simulink model "STFTDiffWindowSizes"  (R2021b)
settings: Solver=VariableStepAuto  StartTime=0.0  StopTime=2048*15/fs  RelTol=1e-3
InitFcn:
  | f = 12.288e6;
  | fs = 153.6e6;
  | N1 = 256;
  | N2 = 512;
  | N3 = 1024;
  | N4 = 2048;
  | N5 = 4096;
  | n1 = 0:N1-1;
  | n2 = 0:N2-1;
  | n3 = 0:N3-1;
  | n4 = 0:N4-1;
  | n5 = 0:N5-1;
  | Hamming1 = 0.54 - 0.46 * cos(2*pi*n1/N1);
  | Hamming2 = 0.54 - 0.46 * cos(2*pi*n2/N2);
  | Hamming3 = 0.54 - 0.46 * cos(2*pi*n3/N3);
  | Hamming4 = 0.54 - 0.46 * cos(2*pi*n4/N4);
  | Hamming5 = 0.54 - 0.46 * cos(2*pi*n5/N5);
  | Hanning1 = 0.5 * (1 + cos(2*pi*n1/N1));
  | Hanning2 = 0.5 * (1 + cos(2*pi*n2/N2));
  | Hanning3 = 0.5 * (1 + cos(2*pi*n3/N3));
  | Hanning4 = 0.5 * (1 + cos(2*pi*n4/N4));
  | Hanning5 = 0.5 * (1 + cos(2*pi*n5/N5));
  | Norm_Ham1 = sum(Hamming1);
  | Norm_Ham2 = sum(Hamming2);
  | Norm_Ham3 = sum(Hamming3);
  | Norm_Ham4 = sum(Hamming4);
  | Norm_Ham5 = sum(Hamming5);
  | Norm_Han1 = sum(Hanning1);
  | Norm_Han2 = sum(Hanning2);
  | Norm_Han3 = sum(Hanning3);
  | Norm_Han4 = sum(Hanning4);
  | Norm_Han5 = sum(Hanning5);
undefined symbols (not defined in the file): AXI4, Lite, Norm_Ham, Norm_Han
libraries: hdlBasic x321, hdlDSPIP x10, hdlsllib x1, vmcUtilities x1
(part 3 of 3)

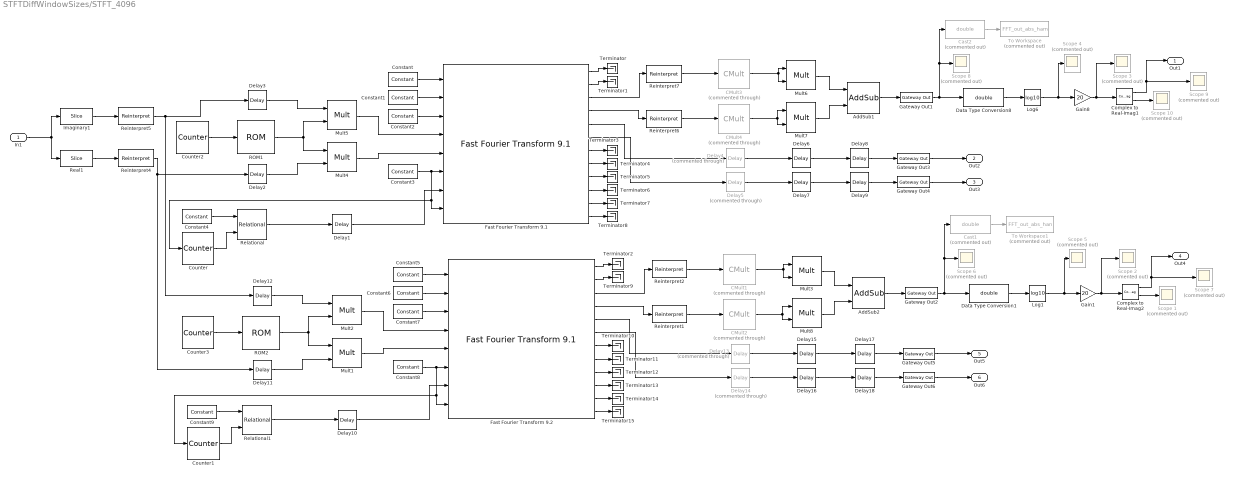
== system STFTDiffWindowSizes/STFT_4096 ==
  In1 : Inport
  AddSub1 : hdlBasic/AddSub  mode=Addition  use_carryin=off  use_carryout=off  en=off  latency=1  precision=User Defined  arith_type=Unsigned  n_bits=32  bin_pt=30  quantization=Truncate  overflow=Saturate  use_behavioral_HDL=off  hw_selection=Fabric  pipelined=off  XmcBlockStatus=1  maskContainerNames=tabcontainer1  block_type=addsub  block_config=sysgen:Addsub_config
  AddSub2 : hdlBasic/AddSub  mode=Addition  use_carryin=off  use_carryout=off  en=off  latency=1  precision=User Defined  arith_type=Unsigned  n_bits=32  bin_pt=30  quantization=Truncate  overflow=Saturate  use_behavioral_HDL=off  hw_selection=Fabric  pipelined=off  XmcBlockStatus=1  maskContainerNames=tabcontainer1  block_type=addsub  block_config=sysgen:Addsub_config
  CMult1 : hdlBasic/CMult  Commented=through  const=1/Norm_Han  gui_display_data_type=Fixed-point  const_n_bits=32  const_bin_pt=31  float_type=Single  exp_bits=8  fraction_bits=24  en=off  latency=3  precision=User Defined  arith_type=Unsigned  n_bits=32  bin_pt=31  quantization=Truncate  overflow=Saturate  use_behavioral_HDL=off  mem_type=Distributed RAM  pipeline=off  XmcBlockStatus=1  maskContainerNames=tabcontainer1  block_type=cmult  block_config=sysgen:CMult_config
      settings: infoedit=[]
  CMult2 : hdlBasic/CMult  Commented=through  const=1/Norm_Han  gui_display_data_type=Fixed-point  const_n_bits=32  const_bin_pt=31  float_type=Single  exp_bits=8  fraction_bits=24  en=off  latency=3  precision=User Defined  arith_type=Unsigned  n_bits=32  bin_pt=31  quantization=Truncate  overflow=Saturate  use_behavioral_HDL=off  mem_type=Distributed RAM  pipeline=off  XmcBlockStatus=1  maskContainerNames=tabcontainer1  block_type=cmult  block_config=sysgen:CMult_config
      settings: infoedit=[]
  CMult3 : hdlBasic/CMult  Commented=through  const=1/Norm_Ham  gui_display_data_type=Fixed-point  const_n_bits=32  const_bin_pt=31  float_type=Single  exp_bits=8  fraction_bits=24  en=off  latency=3  precision=User Defined  arith_type=Unsigned  n_bits=32  bin_pt=31  quantization=Truncate  overflow=Saturate  use_behavioral_HDL=off  mem_type=Distributed RAM  pipeline=off  XmcBlockStatus=1  maskContainerNames=tabcontainer1  block_type=cmult  block_config=sysgen:CMult_config
      settings: infoedit=[]
  CMult4 : hdlBasic/CMult  Commented=through  const=1/Norm_Ham  gui_display_data_type=Fixed-point  const_n_bits=32  const_bin_pt=31  float_type=Single  exp_bits=8  fraction_bits=24  en=off  latency=3  precision=User Defined  arith_type=Unsigned  n_bits=32  bin_pt=31  quantization=Truncate  overflow=Saturate  use_behavioral_HDL=off  mem_type=Distributed RAM  pipeline=off  XmcBlockStatus=1  maskContainerNames=tabcontainer1  block_type=cmult  block_config=sysgen:CMult_config
      settings: infoedit=[]
  Cast1 : DataTypeConversion  Commented=on  OutDataTypeStr=double
  Cast2 : DataTypeConversion  Commented=on  OutDataTypeStr=double
  Complex to Real-Imag1 : ComplexToRealImag
  Complex to Real-Imag2 : ComplexToRealImag
  Constant : hdlBasic/Constant  const=0  gui_display_data_type=Fixed-point  arith_type=Unsigned  n_bits=12  bin_pt=0  preci_type=Single  exp_width=8  frac_width=24  explicit_period=on  period=1/fs  XmcBlockStatus=1  maskContainerNames=tabcontainer1  block_type=constant  block_config=sysgen:Constant_config
  Constant1 : hdlBasic/Constant  const=0  gui_display_data_type=Fixed-point  arith_type=Unsigned  n_bits=1  bin_pt=0  preci_type=Single  exp_width=8  frac_width=24  explicit_period=on  period=1/fs  XmcBlockStatus=1  maskContainerNames=tabcontainer1  block_type=constant  block_config=sysgen:Constant_config
  Constant2 : hdlBasic/Constant  const=0  gui_display_data_type=Boolean  arith_type=Boolean  n_bits=1  bin_pt=0  preci_type=Single  exp_width=8  frac_width=24  explicit_period=on  period=1/fs  XmcBlockStatus=1  maskContainerNames=tabcontainer1  block_type=constant  block_config=sysgen:Constant_config
  Constant3 : hdlBasic/Constant  const=1  gui_display_data_type=Boolean  arith_type=Boolean  n_bits=1  bin_pt=0  preci_type=Single  exp_width=8  frac_width=24  explicit_period=on  period=1/fs  XmcBlockStatus=1  maskContainerNames=tabcontainer1  block_type=constant  block_config=sysgen:Constant_config
  Constant4 : hdlBasic/Constant  const=N5-1  gui_display_data_type=Fixed-point  arith_type=Unsigned  n_bits=12  bin_pt=0  preci_type=Single  exp_width=8  frac_width=24  explicit_period=on  period=1/fs  XmcBlockStatus=1  maskContainerNames=tabcontainer1  block_type=constant  block_config=sysgen:Constant_config
  Constant5 : hdlBasic/Constant  const=0  gui_display_data_type=Fixed-point  arith_type=Unsigned  n_bits=12  bin_pt=0  preci_type=Single  exp_width=8  frac_width=24  explicit_period=on  period=1/fs  XmcBlockStatus=1  maskContainerNames=tabcontainer1  block_type=constant  block_config=sysgen:Constant_config
  Constant6 : hdlBasic/Constant  const=0  gui_display_data_type=Fixed-point  arith_type=Unsigned  n_bits=1  bin_pt=0  preci_type=Single  exp_width=8  frac_width=24  explicit_period=on  period=1/fs  XmcBlockStatus=1  maskContainerNames=tabcontainer1  block_type=constant  block_config=sysgen:Constant_config
  Constant7 : hdlBasic/Constant  const=0  gui_display_data_type=Boolean  arith_type=Boolean  n_bits=1  bin_pt=0  preci_type=Single  exp_width=8  frac_width=24  explicit_period=on  period=1/fs  XmcBlockStatus=1  maskContainerNames=tabcontainer1  block_type=constant  block_config=sysgen:Constant_config
  Constant8 : hdlBasic/Constant  const=1  gui_display_data_type=Boolean  arith_type=Boolean  n_bits=1  bin_pt=0  preci_type=Single  exp_width=8  frac_width=24  explicit_period=on  period=1/fs  XmcBlockStatus=1  maskContainerNames=tabcontainer1  block_type=constant  block_config=sysgen:Constant_config
  Constant9 : hdlBasic/Constant  const=N5-1  gui_display_data_type=Fixed-point  arith_type=Unsigned  n_bits=12  bin_pt=0  preci_type=Single  exp_width=8  frac_width=24  explicit_period=on  period=1/fs  XmcBlockStatus=1  maskContainerNames=tabcontainer1  block_type=constant  block_config=sysgen:Constant_config
  Counter : hdlBasic/Counter  cnt_type=Count limited  cnt_to=N5-1  operation=Up  start_count=0  cnt_by_val=1  arith_type=Unsigned  n_bits=12  bin_pt=0  load_pin=off  rst=off  en=on  explicit_period=Explicit  period=1/fs  use_behavioral_HDL=off  implementation=Fabric  XmcBlockStatus=1  maskContainerNames=group1  block_type=counter  block_config=sysgen:Counter_config
  Counter1 : hdlBasic/Counter  cnt_type=Count limited  cnt_to=N5-1  operation=Up  start_count=0  cnt_by_val=1  arith_type=Unsigned  n_bits=12  bin_pt=0  load_pin=off  rst=off  en=on  explicit_period=Explicit  period=1/fs  use_behavioral_HDL=off  implementation=Fabric  XmcBlockStatus=1  maskContainerNames=group1  block_type=counter  block_config=sysgen:Counter_config
  Counter2 : hdlBasic/Counter  cnt_type=Count limited  cnt_to=N5-1  operation=Up  start_count=0  cnt_by_val=1  arith_type=Unsigned  n_bits=12  bin_pt=0  load_pin=off  rst=off  en=off  explicit_period=Explicit  period=1/fs  use_behavioral_HDL=off  implementation=Fabric  XmcBlockStatus=1  maskContainerNames=group1  block_type=counter  block_config=sysgen:Counter_config
  Counter3 : hdlBasic/Counter  cnt_type=Count limited  cnt_to=N5-1  operation=Up  start_count=0  cnt_by_val=1  arith_type=Unsigned  n_bits=12  bin_pt=0  load_pin=off  rst=off  en=off  explicit_period=Explicit  period=1/fs  use_behavioral_HDL=off  implementation=Fabric  XmcBlockStatus=1  maskContainerNames=group1  block_type=counter  block_config=sysgen:Counter_config
  Data Type Conversion1 : DataTypeConversion  OutDataTypeStr=double  SaturateOnIntegerOverflow=on
  Data Type Conversion8 : DataTypeConversion  OutDataTypeStr=double  SaturateOnIntegerOverflow=on
  Delay{1,6..7,10,15..16} (6 alike) : hdlBasic/Delay  rst=off  en=off  latency=3  reg_retiming=off  XmcBlockStatus=1  maskContainerNames=group1  block_type=delay  block_config=sysgen:Delay_config
  Delay{2..3,8..9,11..12,17..18} (8 alike) : hdlBasic/Delay  rst=off  en=off  latency=1  reg_retiming=off  XmcBlockStatus=1  maskContainerNames=group1  block_type=delay  block_config=sysgen:Delay_config
  Delay{4..5,13..14} (4 alike) : hdlBasic/Delay  Commented=through  rst=off  en=off  latency=3  reg_retiming=off  XmcBlockStatus=1  maskContainerNames=group1  block_type=delay  block_config=sysgen:Delay_config
  Fast Fourier Transform 9.1 : hdlDSPIP/Fast Fourier Transform 9.1   transform_length=4096  target_clock_frequency=200  target_data_throughput=50  implementation_options=pipelined_streaming_io  run_time_configurable_transform_length=off  phase_factor_width=16  scaling_options=scaled  rounding_modes=truncation  aclken=off  aresetn=off  output_ordering=natural_order  cyclic_prefix_insertion=off  throttle_scheme=nonrealtime  xk_index=off  ovflo=off  trim_axipin_name=on  memory_options_data=block_ram  memory_options_phase_factors=block_ram  number_of_stages_using_block_ram_for_data_and_phase_factors=6  memory_options_reorder=block_ram  memory_options_hybrid=off  complex_mult_type=use_mults_resources  butterfly_type=use_luts  simulation_type=hybrid_sim  simulation_model=sysgen:xfftv9_cmodel  data_path_portlist={ 's_axis_data_tdata', 'm_axis_data_tdata', 'm_axis_status_tdata', 'event_fft_overflow' }  channels=1  input_ordering=natural_order  input_width=16  ip_name=Fast Fourier Transform  ip_version=9.1  dsptool_ready=true  ipcore_usecache=true  ipcore_useipmodelcache=true  wrapper_available=true  port_translation_map={ 'aclken' => 'en', 'aresetn' => 'rst'}  data_format=fixed_point  XmcBlockStatus=1  maskContainerNames=tabcontainer1  block_type=xfft_v9_1  block_config=sysgen:rodinimport_config
  Fast Fourier Transform 9.2 : hdlDSPIP/Fast Fourier Transform 9.1   transform_length=4096  target_clock_frequency=200  target_data_throughput=50  implementation_options=pipelined_streaming_io  run_time_configurable_transform_length=off  phase_factor_width=16  scaling_options=scaled  rounding_modes=truncation  aclken=off  aresetn=off  output_ordering=natural_order  cyclic_prefix_insertion=off  throttle_scheme=nonrealtime  xk_index=off  ovflo=off  trim_axipin_name=on  memory_options_data=block_ram  memory_options_phase_factors=block_ram  number_of_stages_using_block_ram_for_data_and_phase_factors=6  memory_options_reorder=block_ram  memory_options_hybrid=off  complex_mult_type=use_mults_resources  butterfly_type=use_luts  simulation_type=hybrid_sim  simulation_model=sysgen:xfftv9_cmodel  data_path_portlist={ 's_axis_data_tdata', 'm_axis_data_tdata', 'm_axis_status_tdata', 'event_fft_overflow' }  channels=1  input_ordering=natural_order  input_width=16  ip_name=Fast Fourier Transform  ip_version=9.1  dsptool_ready=true  ipcore_usecache=true  ipcore_useipmodelcache=true  wrapper_available=true  port_translation_map={ 'aclken' => 'en', 'aresetn' => 'rst'}  data_format=fixed_point  XmcBlockStatus=1  maskContainerNames=tabcontainer1  block_type=xfft_v9_1  block_config=sysgen:rodinimport_config
  Gain1 : Gain  Gain=20
  Gain8 : Gain  Gain=20
  Gateway Out1 : hdlBasic/Gateway Out  inherit_from_input=on  hdl_port=on  rows=1  columns=1  UseAsDAC=off  DACChannel='1'  interface=AXI4-Lite  automatic_assignment=on  address_offset=hex2dec('00')  intf_name=''  intf_description=''  timing_constraint=None  locs_specified=off  LOCs={}  io_standard={}  XmcBlockStatus=1  maskContainerNames=group4  block_type=gatewayout  block_config=sysgen:gateway_out_config  block_width_w=590  block_height_w=620  block_width=620  block_height=750
  Gateway Out2 : hdlBasic/Gateway Out  inherit_from_input=on  hdl_port=on  rows=1  columns=1  UseAsDAC=off  DACChannel='1'  interface=AXI4-Lite  automatic_assignment=on  address_offset=hex2dec('00')  intf_name=''  intf_description=''  timing_constraint=None  locs_specified=off  LOCs={}  io_standard={}  XmcBlockStatus=1  maskContainerNames=group4  block_type=gatewayout  block_config=sysgen:gateway_out_config  block_width_w=590  block_height_w=620  block_width=620  block_height=750
  Gateway Out{3..6} (4 alike) : hdlBasic/Gateway Out  inherit_from_input=off  hdl_port=on  rows=1  columns=1  UseAsDAC=off  DACChannel='1'  interface=AXI4-Lite  automatic_assignment=on  address_offset=hex2dec('00')  intf_name=''  intf_description=''  timing_constraint=None  locs_specified=off  LOCs={}  io_standard={}  XmcBlockStatus=1  maskContainerNames=group4  block_type=gatewayout  block_config=sysgen:gateway_out_config  block_width_w=590  block_height_w=620  block_width=620  block_height=750
  Imaginary1 : hdlBasic/Slice  nbits=16  boolean_output=off  mode=Two Bit Locations  bit1=31  base1=LSB of Input  bit0=16  base0=LSB of Input  XmcBlockStatus=1  maskContainerNames=group1  block_type=slice  block_config=sysgen:Slice_config
  Log1 : Math  Operator=log10  OutputSignalType=complex  SaturateOnIntegerOverflow=on
  Log6 : Math  Operator=log10  OutputSignalType=complex  SaturateOnIntegerOverflow=on
  Mult{1..2,4..5} (4 alike) : hdlBasic/Mult  precision=User Defined  arith_type="Signed  (2's comp)"  n_bits=16  bin_pt=15  quantization=Truncate  overflow=Saturate  en=off  latency=3  use_behavioral_HDL=off  opt=Speed  use_embedded=on  optimum_pipeline=off  pipeline=on  use_rpm=on  placement_style=Triangular  XmcBlockStatus=1  maskContainerNames=group1  block_type=mult  block_config=sysgen:Mult_config
  Mult{3,6..8} (4 alike) : hdlBasic/Mult  precision=User Defined  arith_type=Unsigned  n_bits=32  bin_pt=31  quantization=Truncate  overflow=Saturate  en=off  latency=3  use_behavioral_HDL=off  opt=Speed  use_embedded=on  optimum_pipeline=off  pipeline=on  use_rpm=on  placement_style=Triangular  XmcBlockStatus=1  maskContainerNames=group1  block_type=mult  block_config=sysgen:Mult_config
  ROM1 : hdlBasic/ROM  depth=N5  initVector=Hamming5  distributed_mem=Block RAM  rst=off  init_reg=0  en=off  latency=1  gui_display_data_type=Fixed-point  arith_type=Unsigned  n_bits=16  bin_pt=15  preci_type=Single  exp_width=8  frac_width=24  optimize=Area  use_rpm=on  simulation_type=fast_sim  XmcBlockStatus=1  maskContainerNames=tabcontainer1  block_type=sprom  block_config=sysgen:SPROM_config
  ROM2 : hdlBasic/ROM  depth=N5  initVector=Hanning5  distributed_mem=Block RAM  rst=off  init_reg=0  en=off  latency=1  gui_display_data_type=Fixed-point  arith_type=Unsigned  n_bits=16  bin_pt=15  preci_type=Single  exp_width=8  frac_width=24  optimize=Area  use_rpm=on  simulation_type=fast_sim  XmcBlockStatus=1  maskContainerNames=tabcontainer1  block_type=sprom  block_config=sysgen:SPROM_config
  Real1 : hdlBasic/Slice  nbits=16  boolean_output=off  mode=Two Bit Locations  bit1=15  base1=LSB of Input  bit0=0  base0=LSB of Input  XmcBlockStatus=1  maskContainerNames=group1  block_type=slice  block_config=sysgen:Slice_config
  Reinterpret{1..2,6..7} (4 alike) : hdlBasic/Reinterpret  force_arith_type=on  arith_type="Signed  (2's comp)"  force_bin_pt=off  bin_pt=31  XmcBlockStatus=1  maskContainerNames=group1  block_type=reinterpret  block_config=sysgen:Reinterpret_config
  Reinterpret4 : hdlBasic/Reinterpret  force_arith_type=on  arith_type="Signed  (2's comp)"  force_bin_pt=on  bin_pt=14  XmcBlockStatus=1  maskContainerNames=group1  block_type=reinterpret  block_config=sysgen:Reinterpret_config
  Reinterpret5 : hdlBasic/Reinterpret  force_arith_type=on  arith_type="Signed  (2's comp)"  force_bin_pt=on  bin_pt=14  XmcBlockStatus=1  maskContainerNames=group1  block_type=reinterpret  block_config=sysgen:Reinterpret_config
  Relational : hdlBasic/Relational  mode=a=b  op_type=Bool  en=off  latency=1  XmcBlockStatus=1  maskContainerNames=tabcontainer1  block_type=relational  block_config=sysgen:Relational_config
  Relational1 : hdlBasic/Relational  mode=a=b  op_type=Bool  en=off  latency=1  XmcBlockStatus=1  maskContainerNames=tabcontainer1  block_type=relational  block_config=sysgen:Relational_config
  Scope {1..10} (10 alike) : Scope  Commented=on
  Terminator{,1..15} (16 alike) : Terminator
  To Workspace : ToWorkspace  Commented=on  VariableName=FFT_out_abs_ham  SampleTime=-1
      settings: Save2DSignal=2-D array (concatenate along first dimension)
  To Workspace1 : ToWorkspace  Commented=on  VariableName=FFT_out_abs_han  SampleTime=-1
      settings: Save2DSignal=2-D array (concatenate along first dimension)
  Out1 : Outport
  Out2 : Outport  Port=2
  Out3 : Outport  Port=3
  Out4 : Outport  Port=4
  Out5 : Outport  Port=5
  Out6 : Outport  Port=6
  wires:
  Constant2/1 -> Fast Fourier Transform 9.1/3
  Fast Fourier Transform 9.1/5 -> Delay4/1
  Delay8/1 -> Gateway Out3/1
  Constant3/1 -> Fast Fourier Transform 9.1/6, Fast Fourier Transform 9.1/8, Counter/1
  Delay4/1 -> Delay6/1
  Delay7/1 -> Delay9/1
  Delay2/1 -> Mult4/2
  ROM1/1 -> Mult5/2, Mult4/1
  Delay6/1 -> Delay8/1
  Fast Fourier Transform 9.1/3 -> Reinterpret7/1
  Gateway Out1/1 -> Cast2/1, Scope 8/1, Data Type Conversion8/1
  Constant1/1 -> Fast Fourier Transform 9.1/2
  Fast Fourier Transform 9.1/7 -> Terminator3/1
  Fast Fourier Transform 9.1/1 -> Terminator/1
  Fast Fourier Transform 9.1/10 -> Terminator6/1
  Fast Fourier Transform 9.1/12 -> Terminator8/1
  Fast Fourier Transform 9.1/6 -> Delay5/1
  Imaginary1/1 -> Reinterpret5/1
  Constant/1 -> Fast Fourier Transform 9.1/1
  Fast Fourier Transform 9.1/2 -> Terminator1/1
  Delay1/1 -> Fast Fourier Transform 9.1/7
  In1/1 -> Real1/1, Imaginary1/1
  Reinterpret6/1 -> CMult4/1
  Gateway Out3/1 -> Out2/1
  AddSub1/1 -> Gateway Out1/1
  Gateway Out4/1 -> Out3/1
  Fast Fourier Transform 9.1/4 -> Reinterpret6/1
  Delay5/1 -> Delay7/1
  CMult3/1 -> Mult6/1, Mult6/2
  Fast Fourier Transform 9.1/11 -> Terminator7/1
  CMult4/1 -> Mult7/1, Mult7/2
  Mult4/1 -> Fast Fourier Transform 9.1/5
  Complex to Real-Imag1/1 -> Out1/1, Scope 9/1
  Counter/1 -> Relational/2
  Gain8/1 -> Scope 3/1, Complex to Real-Imag1/1
  Log6/1 -> Scope 4/1, Gain8/1
  Mult7/1 -> AddSub1/2
  Reinterpret7/1 -> CMult3/1
  Fast Fourier Transform 9.1/8 -> Terminator4/1
  Complex to Real-Imag1/2 -> Scope 10/1
  Real1/1 -> Reinterpret4/1
  Constant4/1 -> Relational/1
  Data Type Conversion8/1 -> Log6/1
  Counter2/1 -> ROM1/1
  Mult5/1 -> Fast Fourier Transform 9.1/4
  Relational/1 -> Delay1/1
  Mult6/1 -> AddSub1/1
  Cast2/1 -> To Workspace/1
  Delay9/1 -> Gateway Out4/1
  Delay3/1 -> Mult5/1
  Fast Fourier Transform 9.1/9 -> Terminator5/1
  Fast Fourier Transform 9.2/9 -> Terminator12/1
  Delay12/1 -> Mult2/1
  Delay18/1 -> Gateway Out6/1
  Cast1/1 -> To Workspace1/1
  Mult3/1 -> AddSub2/1
  Relational1/1 -> Delay10/1
  Mult2/1 -> Fast Fourier Transform 9.2/4
  Counter3/1 -> ROM2/1
  Data Type Conversion1/1 -> Log1/1
  Constant9/1 -> Relational1/1
  Complex to Real-Imag2/2 -> Scope 1/1
  Fast Fourier Transform 9.2/8 -> Terminator11/1
  Reinterpret2/1 -> CMult1/1
  Reinterpret4/1 -> Delay11/1, Delay2/1
  Mult8/1 -> AddSub2/2
  Log1/1 -> Gain1/1, Scope 5/1
  Gain1/1 -> Complex to Real-Imag2/1, Scope 2/1
  Counter1/1 -> Relational1/2
  Complex to Real-Imag2/1 -> Scope 7/1, Out4/1
  Mult1/1 -> Fast Fourier Transform 9.2/5
  CMult2/1 -> Mult8/2, Mult8/1
  Reinterpret5/1 -> Delay12/1, Delay3/1
  Fast Fourier Transform 9.2/11 -> Terminator14/1
  CMult1/1 -> Mult3/2, Mult3/1
  Delay14/1 -> Delay16/1
  Fast Fourier Transform 9.2/4 -> Reinterpret1/1
  Gateway Out6/1 -> Out6/1
  AddSub2/1 -> Gateway Out2/1
  Gateway Out5/1 -> Out5/1
  Reinterpret1/1 -> CMult2/1
  Delay10/1 -> Fast Fourier Transform 9.2/7
  Fast Fourier Transform 9.2/2 -> Terminator9/1
  Constant5/1 -> Fast Fourier Transform 9.2/1
  Fast Fourier Transform 9.2/6 -> Delay14/1
  Fast Fourier Transform 9.2/12 -> Terminator15/1
  Fast Fourier Transform 9.2/10 -> Terminator13/1
  Fast Fourier Transform 9.2/1 -> Terminator2/1
  Fast Fourier Transform 9.2/7 -> Terminator10/1
  Constant6/1 -> Fast Fourier Transform 9.2/2
  Gateway Out2/1 -> Data Type Conversion1/1, Scope 6/1, Cast1/1
  Fast Fourier Transform 9.2/3 -> Reinterpret2/1
  Delay15/1 -> Delay17/1
  ROM2/1 -> Mult1/1, Mult2/2
  Delay11/1 -> Mult1/2
  Delay16/1 -> Delay18/1
  Delay13/1 -> Delay15/1
  Constant8/1 -> Counter1/1, Fast Fourier Transform 9.2/8, Fast Fourier Transform 9.2/6
  Delay17/1 -> Gateway Out5/1
  Fast Fourier Transform 9.2/5 -> Delay13/1
  Constant7/1 -> Fast Fourier Transform 9.2/3

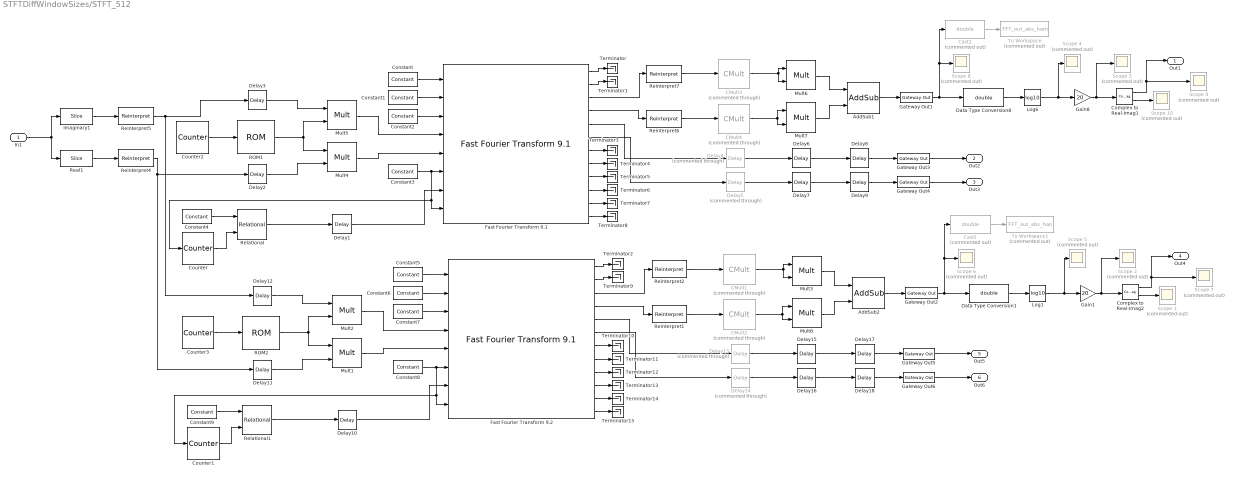
== system STFTDiffWindowSizes/STFT_512 ==
  In1 : Inport
  AddSub1 : hdlBasic/AddSub  mode=Addition  use_carryin=off  use_carryout=off  en=off  latency=1  precision=User Defined  arith_type=Unsigned  n_bits=32  bin_pt=30  quantization=Truncate  overflow=Saturate  use_behavioral_HDL=off  hw_selection=Fabric  pipelined=off  XmcBlockStatus=1  maskContainerNames=tabcontainer1  block_type=addsub  block_config=sysgen:Addsub_config
  AddSub2 : hdlBasic/AddSub  mode=Addition  use_carryin=off  use_carryout=off  en=off  latency=1  precision=User Defined  arith_type=Unsigned  n_bits=32  bin_pt=30  quantization=Truncate  overflow=Saturate  use_behavioral_HDL=off  hw_selection=Fabric  pipelined=off  XmcBlockStatus=1  maskContainerNames=tabcontainer1  block_type=addsub  block_config=sysgen:Addsub_config
  CMult1 : hdlBasic/CMult  Commented=through  const=1/Norm_Han  gui_display_data_type=Fixed-point  const_n_bits=32  const_bin_pt=31  float_type=Single  exp_bits=8  fraction_bits=24  en=off  latency=3  precision=User Defined  arith_type=Unsigned  n_bits=32  bin_pt=31  quantization=Truncate  overflow=Saturate  use_behavioral_HDL=off  mem_type=Distributed RAM  pipeline=off  XmcBlockStatus=1  maskContainerNames=tabcontainer1  block_type=cmult  block_config=sysgen:CMult_config
      settings: infoedit=[]
  CMult2 : hdlBasic/CMult  Commented=through  const=1/Norm_Han  gui_display_data_type=Fixed-point  const_n_bits=32  const_bin_pt=31  float_type=Single  exp_bits=8  fraction_bits=24  en=off  latency=3  precision=User Defined  arith_type=Unsigned  n_bits=32  bin_pt=31  quantization=Truncate  overflow=Saturate  use_behavioral_HDL=off  mem_type=Distributed RAM  pipeline=off  XmcBlockStatus=1  maskContainerNames=tabcontainer1  block_type=cmult  block_config=sysgen:CMult_config
      settings: infoedit=[]
  CMult3 : hdlBasic/CMult  Commented=through  const=1/Norm_Ham  gui_display_data_type=Fixed-point  const_n_bits=32  const_bin_pt=31  float_type=Single  exp_bits=8  fraction_bits=24  en=off  latency=3  precision=User Defined  arith_type=Unsigned  n_bits=32  bin_pt=31  quantization=Truncate  overflow=Saturate  use_behavioral_HDL=off  mem_type=Distributed RAM  pipeline=off  XmcBlockStatus=1  maskContainerNames=tabcontainer1  block_type=cmult  block_config=sysgen:CMult_config
      settings: infoedit=[]
  CMult4 : hdlBasic/CMult  Commented=through  const=1/Norm_Ham  gui_display_data_type=Fixed-point  const_n_bits=32  const_bin_pt=31  float_type=Single  exp_bits=8  fraction_bits=24  en=off  latency=3  precision=User Defined  arith_type=Unsigned  n_bits=32  bin_pt=31  quantization=Truncate  overflow=Saturate  use_behavioral_HDL=off  mem_type=Distributed RAM  pipeline=off  XmcBlockStatus=1  maskContainerNames=tabcontainer1  block_type=cmult  block_config=sysgen:CMult_config
      settings: infoedit=[]
  Cast1 : DataTypeConversion  Commented=on  OutDataTypeStr=double
  Cast2 : DataTypeConversion  Commented=on  OutDataTypeStr=double
  Complex to Real-Imag1 : ComplexToRealImag
  Complex to Real-Imag2 : ComplexToRealImag
  Constant : hdlBasic/Constant  const=0  gui_display_data_type=Fixed-point  arith_type=Unsigned  n_bits=10  bin_pt=0  preci_type=Single  exp_width=8  frac_width=24  explicit_period=on  period=1/fs  XmcBlockStatus=1  maskContainerNames=tabcontainer1  block_type=constant  block_config=sysgen:Constant_config
  Constant1 : hdlBasic/Constant  const=0  gui_display_data_type=Fixed-point  arith_type=Unsigned  n_bits=1  bin_pt=0  preci_type=Single  exp_width=8  frac_width=24  explicit_period=on  period=1/fs  XmcBlockStatus=1  maskContainerNames=tabcontainer1  block_type=constant  block_config=sysgen:Constant_config
  Constant2 : hdlBasic/Constant  const=0  gui_display_data_type=Boolean  arith_type=Boolean  n_bits=1  bin_pt=0  preci_type=Single  exp_width=8  frac_width=24  explicit_period=on  period=1/fs  XmcBlockStatus=1  maskContainerNames=tabcontainer1  block_type=constant  block_config=sysgen:Constant_config
  Constant3 : hdlBasic/Constant  const=1  gui_display_data_type=Boolean  arith_type=Boolean  n_bits=1  bin_pt=0  preci_type=Single  exp_width=8  frac_width=24  explicit_period=on  period=1/fs  XmcBlockStatus=1  maskContainerNames=tabcontainer1  block_type=constant  block_config=sysgen:Constant_config
  Constant4 : hdlBasic/Constant  const=N2-1  gui_display_data_type=Fixed-point  arith_type=Unsigned  n_bits=9  bin_pt=0  preci_type=Single  exp_width=8  frac_width=24  explicit_period=on  period=1/fs  XmcBlockStatus=1  maskContainerNames=tabcontainer1  block_type=constant  block_config=sysgen:Constant_config
  Constant5 : hdlBasic/Constant  const=0  gui_display_data_type=Fixed-point  arith_type=Unsigned  n_bits=10  bin_pt=0  preci_type=Single  exp_width=8  frac_width=24  explicit_period=on  period=1/fs  XmcBlockStatus=1  maskContainerNames=tabcontainer1  block_type=constant  block_config=sysgen:Constant_config
  Constant6 : hdlBasic/Constant  const=0  gui_display_data_type=Fixed-point  arith_type=Unsigned  n_bits=1  bin_pt=0  preci_type=Single  exp_width=8  frac_width=24  explicit_period=on  period=1/fs  XmcBlockStatus=1  maskContainerNames=tabcontainer1  block_type=constant  block_config=sysgen:Constant_config
  Constant7 : hdlBasic/Constant  const=0  gui_display_data_type=Boolean  arith_type=Boolean  n_bits=1  bin_pt=0  preci_type=Single  exp_width=8  frac_width=24  explicit_period=on  period=1/fs  XmcBlockStatus=1  maskContainerNames=tabcontainer1  block_type=constant  block_config=sysgen:Constant_config
  Constant8 : hdlBasic/Constant  const=1  gui_display_data_type=Boolean  arith_type=Boolean  n_bits=1  bin_pt=0  preci_type=Single  exp_width=8  frac_width=24  explicit_period=on  period=1/fs  XmcBlockStatus=1  maskContainerNames=tabcontainer1  block_type=constant  block_config=sysgen:Constant_config
  Constant9 : hdlBasic/Constant  const=N2-1  gui_display_data_type=Fixed-point  arith_type=Unsigned  n_bits=9  bin_pt=0  preci_type=Single  exp_width=8  frac_width=24  explicit_period=on  period=1/fs  XmcBlockStatus=1  maskContainerNames=tabcontainer1  block_type=constant  block_config=sysgen:Constant_config
  Counter : hdlBasic/Counter  cnt_type=Count limited  cnt_to=N1-1  operation=Up  start_count=0  cnt_by_val=1  arith_type=Unsigned  n_bits=8  bin_pt=0  load_pin=off  rst=off  en=on  explicit_period=Explicit  period=1/fs  use_behavioral_HDL=off  implementation=Fabric  XmcBlockStatus=1  maskContainerNames=group1  block_type=counter  block_config=sysgen:Counter_config
  Counter1 : hdlBasic/Counter  cnt_type=Count limited  cnt_to=N2-1  operation=Up  start_count=0  cnt_by_val=1  arith_type=Unsigned  n_bits=9  bin_pt=0  load_pin=off  rst=off  en=on  explicit_period=Explicit  period=1/fs  use_behavioral_HDL=off  implementation=Fabric  XmcBlockStatus=1  maskContainerNames=group1  block_type=counter  block_config=sysgen:Counter_config
  Counter2 : hdlBasic/Counter  cnt_type=Count limited  cnt_to=N2-1  operation=Up  start_count=0  cnt_by_val=1  arith_type=Unsigned  n_bits=9  bin_pt=0  load_pin=off  rst=off  en=off  explicit_period=Explicit  period=1/fs  use_behavioral_HDL=off  implementation=Fabric  XmcBlockStatus=1  maskContainerNames=group1  block_type=counter  block_config=sysgen:Counter_config
  Counter3 : hdlBasic/Counter  cnt_type=Count limited  cnt_to=N2-1  operation=Up  start_count=0  cnt_by_val=1  arith_type=Unsigned  n_bits=9  bin_pt=0  load_pin=off  rst=off  en=off  explicit_period=Explicit  period=1/fs  use_behavioral_HDL=off  implementation=Fabric  XmcBlockStatus=1  maskContainerNames=group1  block_type=counter  block_config=sysgen:Counter_config
  Data Type Conversion1 : DataTypeConversion  OutDataTypeStr=double  SaturateOnIntegerOverflow=on
  Data Type Conversion8 : DataTypeConversion  OutDataTypeStr=double  SaturateOnIntegerOverflow=on
  Delay{1,6..7,10,15..16} (6 alike) : hdlBasic/Delay  rst=off  en=off  latency=3  reg_retiming=off  XmcBlockStatus=1  maskContainerNames=group1  block_type=delay  block_config=sysgen:Delay_config
  Delay{2..3,8..9,11..12,17..18} (8 alike) : hdlBasic/Delay  rst=off  en=off  latency=1  reg_retiming=off  XmcBlockStatus=1  maskContainerNames=group1  block_type=delay  block_config=sysgen:Delay_config
  Delay{4..5,13..14} (4 alike) : hdlBasic/Delay  Commented=through  rst=off  en=off  latency=3  reg_retiming=off  XmcBlockStatus=1  maskContainerNames=group1  block_type=delay  block_config=sysgen:Delay_config
  Fast Fourier Transform 9.1 : hdlDSPIP/Fast Fourier Transform 9.1   transform_length=512  target_clock_frequency=200  target_data_throughput=50  implementation_options=pipelined_streaming_io  run_time_configurable_transform_length=off  phase_factor_width=16  scaling_options=scaled  rounding_modes=truncation  aclken=off  aresetn=off  output_ordering=natural_order  cyclic_prefix_insertion=off  throttle_scheme=nonrealtime  xk_index=off  ovflo=off  trim_axipin_name=on  memory_options_data=block_ram  memory_options_phase_factors=block_ram  number_of_stages_using_block_ram_for_data_and_phase_factors=4  memory_options_reorder=block_ram  memory_options_hybrid=off  complex_mult_type=use_mults_resources  butterfly_type=use_luts  simulation_type=hybrid_sim  simulation_model=sysgen:xfftv9_cmodel  data_path_portlist={ 's_axis_data_tdata', 'm_axis_data_tdata', 'm_axis_status_tdata', 'event_fft_overflow' }  channels=1  input_ordering=natural_order  input_width=16  ip_name=Fast Fourier Transform  ip_version=9.1  dsptool_ready=true  ipcore_usecache=true  ipcore_useipmodelcache=true  wrapper_available=true  port_translation_map={ 'aclken' => 'en', 'aresetn' => 'rst'}  data_format=fixed_point  XmcBlockStatus=1  maskContainerNames=tabcontainer1  block_type=xfft_v9_1  block_config=sysgen:rodinimport_config
  Fast Fourier Transform 9.2 : hdlDSPIP/Fast Fourier Transform 9.1   transform_length=512  target_clock_frequency=200  target_data_throughput=50  implementation_options=pipelined_streaming_io  run_time_configurable_transform_length=off  phase_factor_width=16  scaling_options=scaled  rounding_modes=truncation  aclken=off  aresetn=off  output_ordering=natural_order  cyclic_prefix_insertion=off  throttle_scheme=nonrealtime  xk_index=off  ovflo=off  trim_axipin_name=on  memory_options_data=block_ram  memory_options_phase_factors=block_ram  number_of_stages_using_block_ram_for_data_and_phase_factors=4  memory_options_reorder=block_ram  memory_options_hybrid=off  complex_mult_type=use_mults_resources  butterfly_type=use_luts  simulation_type=hybrid_sim  simulation_model=sysgen:xfftv9_cmodel  data_path_portlist={ 's_axis_data_tdata', 'm_axis_data_tdata', 'm_axis_status_tdata', 'event_fft_overflow' }  channels=1  input_ordering=natural_order  input_width=16  ip_name=Fast Fourier Transform  ip_version=9.1  dsptool_ready=true  ipcore_usecache=true  ipcore_useipmodelcache=true  wrapper_available=true  port_translation_map={ 'aclken' => 'en', 'aresetn' => 'rst'}  data_format=fixed_point  XmcBlockStatus=1  maskContainerNames=tabcontainer1  block_type=xfft_v9_1  block_config=sysgen:rodinimport_config
  Gain1 : Gain  Gain=20
  Gain8 : Gain  Gain=20
  Gateway Out1 : hdlBasic/Gateway Out  inherit_from_input=on  hdl_port=on  rows=1  columns=1  UseAsDAC=off  DACChannel='1'  interface=AXI4-Lite  automatic_assignment=on  address_offset=hex2dec('00')  intf_name=''  intf_description=''  timing_constraint=None  locs_specified=off  LOCs={}  io_standard={}  XmcBlockStatus=1  maskContainerNames=group4  block_type=gatewayout  block_config=sysgen:gateway_out_config  block_width_w=590  block_height_w=620  block_width=620  block_height=750
  Gateway Out2 : hdlBasic/Gateway Out  inherit_from_input=on  hdl_port=on  rows=1  columns=1  UseAsDAC=off  DACChannel='1'  interface=AXI4-Lite  automatic_assignment=on  address_offset=hex2dec('00')  intf_name=''  intf_description=''  timing_constraint=None  locs_specified=off  LOCs={}  io_standard={}  XmcBlockStatus=1  maskContainerNames=group4  block_type=gatewayout  block_config=sysgen:gateway_out_config  block_width_w=590  block_height_w=620  block_width=620  block_height=750
  Gateway Out{3..6} (4 alike) : hdlBasic/Gateway Out  inherit_from_input=off  hdl_port=on  rows=1  columns=1  UseAsDAC=off  DACChannel='1'  interface=AXI4-Lite  automatic_assignment=on  address_offset=hex2dec('00')  intf_name=''  intf_description=''  timing_constraint=None  locs_specified=off  LOCs={}  io_standard={}  XmcBlockStatus=1  maskContainerNames=group4  block_type=gatewayout  block_config=sysgen:gateway_out_config  block_width_w=590  block_height_w=620  block_width=620  block_height=750
  Imaginary1 : hdlBasic/Slice  nbits=16  boolean_output=off  mode=Two Bit Locations  bit1=31  base1=LSB of Input  bit0=16  base0=LSB of Input  XmcBlockStatus=1  maskContainerNames=group1  block_type=slice  block_config=sysgen:Slice_config
  Log1 : Math  Operator=log10  OutputSignalType=complex  SaturateOnIntegerOverflow=on
  Log6 : Math  Operator=log10  OutputSignalType=complex  SaturateOnIntegerOverflow=on
  Mult{1..2,4..5} (4 alike) : hdlBasic/Mult  precision=User Defined  arith_type="Signed  (2's comp)"  n_bits=16  bin_pt=15  quantization=Truncate  overflow=Saturate  en=off  latency=3  use_behavioral_HDL=off  opt=Speed  use_embedded=on  optimum_pipeline=off  pipeline=on  use_rpm=on  placement_style=Triangular  XmcBlockStatus=1  maskContainerNames=group1  block_type=mult  block_config=sysgen:Mult_config
  Mult{3,6..8} (4 alike) : hdlBasic/Mult  precision=User Defined  arith_type=Unsigned  n_bits=32  bin_pt=31  quantization=Truncate  overflow=Saturate  en=off  latency=3  use_behavioral_HDL=off  opt=Speed  use_embedded=on  optimum_pipeline=off  pipeline=on  use_rpm=on  placement_style=Triangular  XmcBlockStatus=1  maskContainerNames=group1  block_type=mult  block_config=sysgen:Mult_config
  ROM1 : hdlBasic/ROM  depth=N2  initVector=Hamming2  distributed_mem=Block RAM  rst=off  init_reg=0  en=off  latency=1  gui_display_data_type=Fixed-point  arith_type=Unsigned  n_bits=16  bin_pt=15  preci_type=Single  exp_width=8  frac_width=24  optimize=Area  use_rpm=on  simulation_type=fast_sim  XmcBlockStatus=1  maskContainerNames=tabcontainer1  block_type=sprom  block_config=sysgen:SPROM_config
  ROM2 : hdlBasic/ROM  depth=N2  initVector=Hanning2  distributed_mem=Block RAM  rst=off  init_reg=0  en=off  latency=1  gui_display_data_type=Fixed-point  arith_type=Unsigned  n_bits=16  bin_pt=15  preci_type=Single  exp_width=8  frac_width=24  optimize=Area  use_rpm=on  simulation_type=fast_sim  XmcBlockStatus=1  maskContainerNames=tabcontainer1  block_type=sprom  block_config=sysgen:SPROM_config
  Real1 : hdlBasic/Slice  nbits=16  boolean_output=off  mode=Two Bit Locations  bit1=15  base1=LSB of Input  bit0=0  base0=LSB of Input  XmcBlockStatus=1  maskContainerNames=group1  block_type=slice  block_config=sysgen:Slice_config
  Reinterpret{1..2,6..7} (4 alike) : hdlBasic/Reinterpret  force_arith_type=on  arith_type="Signed  (2's comp)"  force_bin_pt=off  bin_pt=31  XmcBlockStatus=1  maskContainerNames=group1  block_type=reinterpret  block_config=sysgen:Reinterpret_config
  Reinterpret4 : hdlBasic/Reinterpret  force_arith_type=on  arith_type="Signed  (2's comp)"  force_bin_pt=on  bin_pt=14  XmcBlockStatus=1  maskContainerNames=group1  block_type=reinterpret  block_config=sysgen:Reinterpret_config
  Reinterpret5 : hdlBasic/Reinterpret  force_arith_type=on  arith_type="Signed  (2's comp)"  force_bin_pt=on  bin_pt=14  XmcBlockStatus=1  maskContainerNames=group1  block_type=reinterpret  block_config=sysgen:Reinterpret_config
  Relational : hdlBasic/Relational  mode=a=b  op_type=Bool  en=off  latency=1  XmcBlockStatus=1  maskContainerNames=tabcontainer1  block_type=relational  block_config=sysgen:Relational_config
  Relational1 : hdlBasic/Relational  mode=a=b  op_type=Bool  en=off  latency=1  XmcBlockStatus=1  maskContainerNames=tabcontainer1  block_type=relational  block_config=sysgen:Relational_config
  Scope {1..10} (10 alike) : Scope  Commented=on
  Terminator{,1..15} (16 alike) : Terminator
  To Workspace : ToWorkspace  Commented=on  VariableName=FFT_out_abs_ham  SampleTime=-1
      settings: Save2DSignal=2-D array (concatenate along first dimension)
  To Workspace1 : ToWorkspace  Commented=on  VariableName=FFT_out_abs_han  SampleTime=-1
      settings: Save2DSignal=2-D array (concatenate along first dimension)
  Out1 : Outport
  Out2 : Outport  Port=2
  Out3 : Outport  Port=3
  Out4 : Outport  Port=4
  Out5 : Outport  Port=5
  Out6 : Outport  Port=6
  wires:
  Constant7/1 -> Fast Fourier Transform 9.2/3
  Fast Fourier Transform 9.2/5 -> Delay13/1
  Delay17/1 -> Gateway Out5/1
  Constant8/1 -> Fast Fourier Transform 9.2/6, Fast Fourier Transform 9.2/8, Counter1/1
  Delay13/1 -> Delay15/1
  Delay16/1 -> Delay18/1
  Delay11/1 -> Mult1/2
  ROM2/1 -> Mult2/2, Mult1/1
  Delay15/1 -> Delay17/1
  Fast Fourier Transform 9.2/3 -> Reinterpret2/1
  Gateway Out2/1 -> Cast1/1, Scope 6/1, Data Type Conversion1/1
  Constant6/1 -> Fast Fourier Transform 9.2/2
  Fast Fourier Transform 9.2/7 -> Terminator10/1
  Fast Fourier Transform 9.2/1 -> Terminator2/1
  Fast Fourier Transform 9.2/10 -> Terminator13/1
  Fast Fourier Transform 9.2/12 -> Terminator15/1
  Fast Fourier Transform 9.2/6 -> Delay14/1
  Constant5/1 -> Fast Fourier Transform 9.2/1
  Fast Fourier Transform 9.2/2 -> Terminator9/1
  Delay10/1 -> Fast Fourier Transform 9.2/7
  Reinterpret1/1 -> CMult2/1
  Gateway Out5/1 -> Out5/1
  AddSub2/1 -> Gateway Out2/1
  Gateway Out6/1 -> Out6/1
  Fast Fourier Transform 9.2/4 -> Reinterpret1/1
  Delay14/1 -> Delay16/1
  CMult1/1 -> Mult3/1, Mult3/2
  Fast Fourier Transform 9.2/11 -> Terminator14/1
  Reinterpret5/1 -> Delay3/1, Delay12/1
  CMult2/1 -> Mult8/1, Mult8/2
  Mult1/1 -> Fast Fourier Transform 9.2/5
  Complex to Real-Imag2/1 -> Out4/1, Scope 7/1
  Counter1/1 -> Relational1/2
  Gain1/1 -> Scope 2/1, Complex to Real-Imag2/1
  Log1/1 -> Scope 5/1, Gain1/1
  Mult8/1 -> AddSub2/2
  Reinterpret4/1 -> Delay2/1, Delay11/1
  Reinterpret2/1 -> CMult1/1
  Fast Fourier Transform 9.2/8 -> Terminator11/1
  Complex to Real-Imag2/2 -> Scope 1/1
  Constant9/1 -> Relational1/1
  Data Type Conversion1/1 -> Log1/1
  Counter3/1 -> ROM2/1
  Mult2/1 -> Fast Fourier Transform 9.2/4
  Relational1/1 -> Delay10/1
  Mult3/1 -> AddSub2/1
  Cast1/1 -> To Workspace1/1
  Delay18/1 -> Gateway Out6/1
  Delay12/1 -> Mult2/1
  Fast Fourier Transform 9.2/9 -> Terminator12/1
  Fast Fourier Transform 9.1/9 -> Terminator5/1
  Delay3/1 -> Mult5/1
  Delay9/1 -> Gateway Out4/1
  Cast2/1 -> To Workspace/1
  Mult6/1 -> AddSub1/1
  Relational/1 -> Delay1/1
  Mult5/1 -> Fast Fourier Transform 9.1/4
  Counter2/1 -> ROM1/1
  Data Type Conversion8/1 -> Log6/1
  Constant4/1 -> Relational/1
  Real1/1 -> Reinterpret4/1
  Complex to Real-Imag1/2 -> Scope 10/1
  Fast Fourier Transform 9.1/8 -> Terminator4/1
  Reinterpret7/1 -> CMult3/1
  Mult7/1 -> AddSub1/2
  Log6/1 -> Gain8/1, Scope 4/1
  Gain8/1 -> Complex to Real-Imag1/1, Scope 3/1
  Counter/1 -> Relational/2
  Complex to Real-Imag1/1 -> Scope 9/1, Out1/1
  Mult4/1 -> Fast Fourier Transform 9.1/5
  CMult4/1 -> Mult7/2, Mult7/1
  Fast Fourier Transform 9.1/11 -> Terminator7/1
  CMult3/1 -> Mult6/2, Mult6/1
  Delay5/1 -> Delay7/1
  Fast Fourier Transform 9.1/4 -> Reinterpret6/1
  Gateway Out4/1 -> Out3/1
  AddSub1/1 -> Gateway Out1/1
  Gateway Out3/1 -> Out2/1
  Reinterpret6/1 -> CMult4/1
  In1/1 -> Imaginary1/1, Real1/1
  Delay1/1 -> Fast Fourier Transform 9.1/7
  Fast Fourier Transform 9.1/2 -> Terminator1/1
  Constant/1 -> Fast Fourier Transform 9.1/1
  Imaginary1/1 -> Reinterpret5/1
  Fast Fourier Transform 9.1/6 -> Delay5/1
  Fast Fourier Transform 9.1/12 -> Terminator8/1
  Fast Fourier Transform 9.1/10 -> Terminator6/1
  Fast Fourier Transform 9.1/1 -> Terminator/1
  Fast Fourier Transform 9.1/7 -> Terminator3/1
  Constant1/1 -> Fast Fourier Transform 9.1/2
  Gateway Out1/1 -> Data Type Conversion8/1, Scope 8/1, Cast2/1
  Fast Fourier Transform 9.1/3 -> Reinterpret7/1
  Delay6/1 -> Delay8/1
  ROM1/1 -> Mult4/1, Mult5/2
  Delay2/1 -> Mult4/2
  Delay7/1 -> Delay9/1
  Delay4/1 -> Delay6/1
  Constant3/1 -> Counter/1, Fast Fourier Transform 9.1/8, Fast Fourier Transform 9.1/6
  Delay8/1 -> Gateway Out3/1
  Fast Fourier Transform 9.1/5 -> Delay4/1
  Constant2/1 -> Fast Fourier Transform 9.1/3
